simulink model "control_model_4"  (R2025b)
settings: Solver=VariableStepAuto  StartTime=0.0  StopTime=300  RelTol=1e-3
values from neighbouring files (symbols this model uses):
  Am = [0 1; -wn^2 -2*zeta*wn]    [Script.m]    (also in main_v2.m = [0 1 0 0; -walpha^2 -2*zeta_alpha*walpha 0 0; 0 0 0 1; 0 0 -; script_plane.m; script_v2.m)
  B = [0; -thrust*static_margin/Iy]    [Script.m]    (also in main_v2.m = [0; Cm_delta/Iy; 0; 0]; script_plane.m = [0; Cm_delta/Iy]; script_v2.m)
  Bm = [0; wn^2]    [Script.m]    (also in main_v2.m = [0; walpha^2; 0; 0]; script_plane.m; script_v2.m)
  c = 3.2    [main_v2.m]    (also in script_plane.m = 3.45)
  Cd0 = 0.02    [main_v2.m]
  Cl0 = 0.1    [main_v2.m]
  Cl_alpha = 5.7    [main_v2.m]
  Cm = [1 0; 0 1]    [Script.m]    (also in main_v2.m = eye(size(Am)); script_plane.m; script_v2.m)
  Cm_0 = -0.8    [main_v2.m]
  Cm_delta = -0.5    [main_v2.m]    (also in script_plane.m = -4.5)
  Cm_q = -12    [main_v2.m]    (also in script_plane.m = -8)
  delta_max = deg2rad(25)    [main_v2.m]    (also in script_plane.m)
  desired_aoa = deg2rad(45)    [main_v2.m]    (also in script_plane.m = deg2rad(20))
  Dm = [0;0]    [Script.m]    (also in main_v2.m = zeros(4, 1); script_plane.m; script_v2.m)
  g = 9.81    [Script.m]    (also in main_v2.m; script_v2.m)
  gain_e = 0    [main_v2.m]    (also in script_plane.m = 5000)
  gain_r = 300    [main_v2.m]    (also in script_plane.m = 50000)
  gain_x = 200    [main_v2.m]    (also in script_plane.m = 50000)
  Iy = 5    [Script.m]    (also in main_v2.m = 160000; script_plane.m = 70000; script_v2.m)
  K = 1/2 *rho * S *c    (= 58.8)    [main_v2.m]    (also in script_plane.m = 1908126.5175)
  k_d1 = 0.045    [main_v2.m]
  k_d2 = 0.08    [main_v2.m]
  kl = 3    [main_v2.m]
  Kr = wn^2/(-thrust*static_margin/Iy)    (= -0.0208333333333)    [Script.m]    (also in main_v2.m = 0; script_plane.m = -0.18; script_v2.m)
  Kx = ((Am-A)/B.').'    [Script.m]    (also in main_v2.m = [0 0 0 0]; script_plane.m = [0.21 0.05]; script_v2.m)
  mass = 15    [Script.m]    (also in main_v2.m = 9000; script_plane.m = 12000; script_v2.m)
  P = lyap(Am',Q)    [Script.m]    (also in main_v2.m; script_plane.m)
  rate_of_change = 4    [main_v2.m]
  rate_of_freeze_angle = 0.8    [main_v2.m]
  rate_of_freeze_rate = 2    [main_v2.m]
  rho = 1.225    [main_v2.m]    (also in script_plane.m)
  S = 30    [main_v2.m]    (also in script_plane.m = 27.87)
  sigma_r = 0.0003    [main_v2.m]    (also in script_plane.m = 1e-05)
  sigma_w = 0.0003    [main_v2.m]    (also in script_plane.m = 1e-05)
  sigma_x = 0.0003    [main_v2.m]    (also in script_plane.m = 1e-05)
  speed = 180    [main_v2.m]    (also in script_plane.m)
  thrust = 6000    [Script.m]    (also in main_v2.m = 160000; script_v2.m)
  W = [0 0 0 0]    [main_v2.m]
libraries: simulink_extras x17, simulink x2, slctrl_adaptive x1
settings Model: Creator=marti  LastModifiedBy=marti
settings SolverCC: ZeroCrossAlgorithm=Adaptive
settings DebuggingCC: IgnoredZcDiagnostic=none

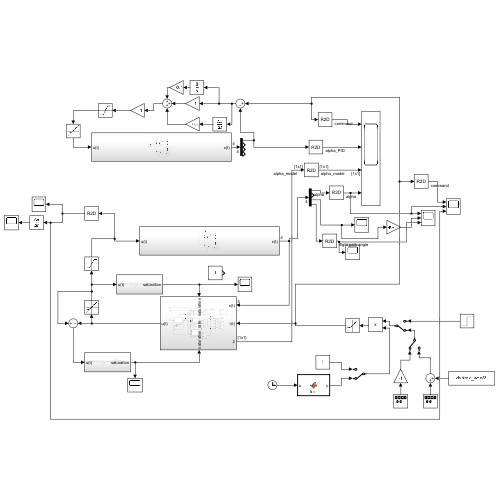
[thumbnail: Simulink's stored preview of the top-level diagram]
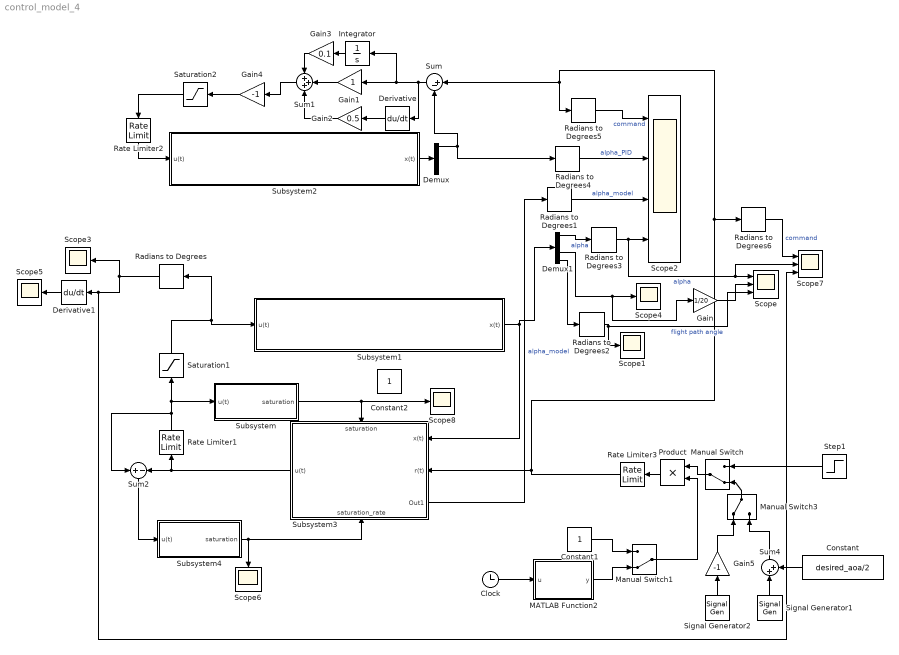
== system control_model_4 ==
  Clock : Clock
  Constant : Constant  Value=desired_aoa/2
  Constant1 : Constant
  Constant2 : Constant
  Demux : Demux
  Demux1 : Demux
  Derivative : Derivative
  Derivative1 : Derivative
  Gain : Gain  Gain=1/20
  Gain1 : Gain
  Gain2 : Gain  Gain=0.5
  Gain3 : Gain  Gain=0.1
  Gain4 : Gain  Gain=-1
  Gain5 : Gain  Gain=-1
  Integrator : Integrator
  MATLAB Function2 : MATLAB Function  TreatAsAtomicUnit=on
  Manual Switch : ManualSwitch  CurrentSetting=0
  Manual Switch1 : ManualSwitch  CurrentSetting=0
  Manual Switch3 : ManualSwitch
  Product : Product
  Radians to Degrees{,1..6} (7 alike) : simulink_extras/Transformations/Radians to Degrees
  Rate Limiter1 : RateLimiter  RisingSlewLimit=deg2rad(60)  FallingSlewLimit=-deg2rad(60)  SampleTimeMode=inherited
  Rate Limiter2 : RateLimiter  RisingSlewLimit=deg2rad(60)  FallingSlewLimit=-deg2rad(60)  SampleTimeMode=inherited
  Rate Limiter3 : RateLimiter  RisingSlewLimit=deg2rad(50)  FallingSlewLimit=-deg2rad(50)  SampleTimeMode=inherited
  Saturation1 : Saturate  UpperLimit=delta_max  LowerLimit=-delta_max  ZeroCross=off
  Saturation2 : Saturate  UpperLimit=delta_max  LowerLimit=-delta_max  ZeroCross=off
  Scope : Scope  NumInputPorts=3
      settings: ActiveDisplayYMinimum=-57.288074409345953  ActiveDisplayYMaximum=57.41030738577799  DataLoggingVariableName=ScopeData3
  Scope{1,3..6,8} (6 alike) : Scope
      Scope1 settings: ActiveDisplayYMinimum=-6.2979573477285218  ActiveDisplayYMaximum=52.72463637167975  DataLoggingVariableName=ScopeData2
      Scope3 settings: ActiveDisplayYMinimum=-31.25  ActiveDisplayYMaximum=31.25  DataLoggingVariableName=ScopeData16
      Scope4 settings: ActiveDisplayYMinimum=134.59247110443181  ActiveDisplayYMaximum=588.66776006011389  DataLoggingVariableName=ScopeData13
      Scope5 settings: ActiveDisplayYMinimum=-135.49485335885979  ActiveDisplayYMaximum=116.59818871809171  DataLoggingVariableName=ScopeData17
      Scope6 settings: ActiveDisplayYMinimum=-0.12499999999999997  ActiveDisplayYMaximum=1.125  DataLoggingVariableName=ScopeData12
      Scope8 settings: ActiveDisplayYMinimum=-0.1187909152069436  ActiveDisplayYMaximum=1.1243100993994897  DataLoggingVariableName=ScopeData18
  Scope2 : Scope  NumInputPorts=4
      settings: ActiveDisplayYMinimum=-78.018833846939785  ActiveDisplayYMaximum=59.661096228054994  DataLoggingVariableName=ScopeData15
  Scope7 : Scope  NumInputPorts=3
      settings: ActiveDisplayYMinimum=-1  ActiveDisplayYMaximum=1  DataLoggingVariableName=ScopeData14
  Signal Generator1 : SignalGenerator  WaveForm=square  Amplitude=desired_aoa/2  Frequency=0.1  Units=rad/sec
  Signal Generator2 : SignalGenerator  WaveForm=square  Amplitude=desired_aoa  Frequency=0.1  Units=rad/sec
  Step1 : Step  Time=31.3  After=desired_aoa  SampleTime=0
  Subsystem : Subsystem
  Subsystem1 : Subsystem
  Subsystem2 : Subsystem
  Subsystem3 : Subsystem
      settings: PortSchema="{\"entries\":[{\"content\":{\"sides\":[{\"content\":{\"connectorIds\":[\"Out2\",\"In1\",\"In2\"]},\"type\":\"ConnectorPlacement.EquallySpacedRectSide\",\"uuid\":\"2a5405b8-f474-466f-9064-f86b75893dd0\"},{\"content\":{\"connectorIds\":[\"Out1\"],\"side\":\"RIGHT\"},\"type\":\"ConnectorPlacement.EquallySpacedRectSide\",\"uuid\":\"ad673661-f4e9-494b-83cc-7452eec3fe31\"},{\"content\":{\"connectorIds\":[\"In3\"],\"side\":\"TOP\"},\"type\":\"ConnectorPlacement.EquallySpacedRectSide\",\"uuid\":\"21a76317-3288-4ff3-bd02-68708e86e3a8\"},{\"content\":{\"connectorIds\":[\"In4\"],\"side\":\"BOTTOM\"},\"type\":\"ConnectorPlacement.EquallySpacedRectSide\",\"uuid\":\"06318006-2373-43e5-8136-a784e8462fed\"}]},\"type\":\"ConnectorPlacement.EquallySpacedConnector\",\"uuid\":\"fc0ce599-928f-4c66-9629-0b98f2391e21\"}],\"packageUris\":[\"http://schema.mathworks.com/mf0/Connector/R2020b\"],\"version\":\"1.0\"}"
  Subsystem4 : Subsystem
  Sum : Sum  Inputs=|+-
  Sum1 : Sum  Inputs=+++
  Sum2 : Sum  Inputs=+|-
  Sum4 : Sum  Inputs=|++
  wires:
  Subsystem1/1(x(t)) -> Demux1/1, Subsystem3/2(x(t))
  Radians to Degrees3/1 -> Scope7/2, Scope/1, Scope2/4  "alpha"
  Radians to Degrees4/1 -> Scope2/2  "alpha_PID"
  Signal Generator1/1 -> Sum4/1
  Derivative1/1 -> Scope5/1
  Subsystem3/1(u(t)) -> Sum2/2, Rate Limiter1/1
  Subsystem4/1(saturation) -> Subsystem3/3(saturation_rate), Scope6/1
  Subsystem3/2(Out1) -> Radians to Degrees1/1  "alpha_model"
  Saturation1/1 -> Subsystem1/1(u(t)), Radians to Degrees/1
  Radians to Degrees1/1 -> Scope2/3  "alpha_model"
  Constant/1 -> Sum4/2
  Manual Switch3/1 -> Manual Switch/2
  Sum2/1 -> Subsystem4/1(u(t))
  Rate Limiter3/1 -> Subsystem3/1(r(t)), Radians to Degrees5/1, Sum/1, Radians to Degrees6/1
  Radians to Degrees5/1 -> Scope2/1  "command"
  Radians to Degrees/1 -> Scope7/3, Derivative1/1, Scope3/1
  Sum4/1 -> Manual Switch3/2
  Demux1/3 -> Gain/1, Scope4/1
  Radians to Degrees2/1 -> Scope1/1, Scope/3  "flight path angle"
  Clock/1 -> MATLAB Function2/1(u)
  Manual Switch/1 -> Product/1
  Product/1 -> Rate Limiter3/1
  Demux1/1 -> Radians to Degrees3/1  "alpha"
  Demux1/4 -> Radians to Degrees2/1
  Step1/1 -> Manual Switch/1
  Constant1/1 -> Manual Switch1/1
  MATLAB Function2/1(y) -> Manual Switch1/2
  Manual Switch1/1 -> Product/2
  Gain/1 -> Scope/2
  Subsystem/1(saturation) -> Scope8/1, Subsystem3/4(saturation)
  Sum/1 -> Derivative/1, Integrator/1, Gain1/1
  Subsystem2/1(x(t)) -> Demux/1
  Demux/1 -> Sum/2, Radians to Degrees4/1
  Gain1/1 -> Sum1/2
  Gain2/1 -> Sum1/3
  Integrator/1 -> Gain3/1
  Gain3/1 -> Sum1/1
  Derivative/1 -> Gain2/1
  Gain4/1 -> Saturation2/1
  Sum1/1 -> Gain4/1
  Saturation2/1 -> Rate Limiter2/1
  Rate Limiter2/1 -> Subsystem2/1(u(t))
  Rate Limiter1/1 -> Sum2/1, Saturation1/1, Subsystem/1(u(t))
  Signal Generator2/1 -> Gain5/1
  Gain5/1 -> Manual Switch3/1
  Radians to Degrees6/1 -> Scope7/1  "command"

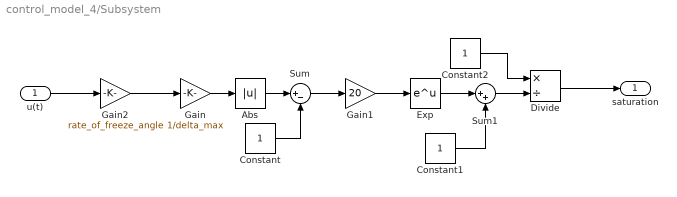
== system control_model_4/Subsystem ==
  u(t) : Inport
  Abs : Abs  SaturateOnIntegerOverflow=off
  Constant : Constant
  Constant1 : Constant
  Constant2 : Constant
  Divide : Product  Inputs=*/
  Exp : Math
  Gain : Gain  Gain=1/delta_max
  Gain1 : Gain  Gain=20
  Gain2 : Gain  Gain=rate_of_freeze_angle
  Sum : Sum  Inputs=|+-
  Sum1 : Sum  Inputs=|++
  saturation : Outport
  wires:
  Gain/1 -> Abs/1
  Abs/1 -> Sum/1
  Sum/1 -> Gain1/1
  Constant/1 -> Sum/2
  Gain1/1 -> Exp/1
  Exp/1 -> Sum1/1
  Constant1/1 -> Sum1/2
  Sum1/1 -> Divide/2
  Constant2/1 -> Divide/1
  Divide/1 -> saturation/1
  Gain2/1 -> Gain/1
  u(t)/1 -> Gain2/1

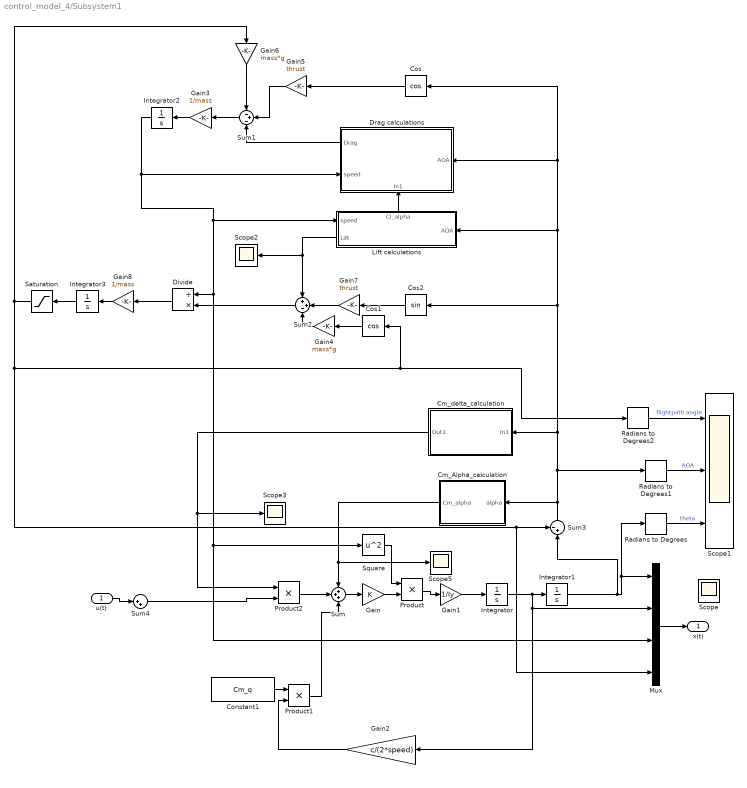
== system control_model_4/Subsystem1 ==
  u(t) : Inport
  Cm_Alpha_calculation : Subsystem
  Cm_delta_calculation : Subsystem
  Constant1 : Constant  Value=Cm_q
  Cos : Trigonometry  Operator=cos
  Cos1 : Trigonometry  Operator=cos
  Cos2 : Trigonometry
  Divide : Product  Inputs=/*
  Drag calculations : Subsystem
      settings: PortSchema="{\"entries\":[{\"content\":{\"sides\":[{\"content\":{\"connectorIds\":[\"Out1\",\"In1\"]},\"type\":\"ConnectorPlacement.EquallySpacedRectSide\",\"uuid\":\"d271dd9c-4b6b-493d-a484-ea343b2a7ea5\"},{\"content\":{\"connectorIds\":[\"In3\"],\"side\":\"RIGHT\"},\"type\":\"ConnectorPlacement.EquallySpacedRectSide\",\"uuid\":\"1c3a3b91-ae49-4f86-b72d-44481f1c47ea\"},{\"content\":{\"side\":\"TOP\"},\"type\":\"ConnectorPlacement.EquallySpacedRectSide\",\"uuid\":\"ad2c4e7a-6e16-439a-a8ce-91c789fc2dda\"},{\"content\":{\"connectorIds\":[\"In2\"],\"side\":\"BOTTOM\"},\"type\":\"ConnectorPlacement.EquallySpacedRectSide\",\"uuid\":\"1d27e3d2-8ebb-4b91-86b1-b9e0cbaba979\"}]},\"type\":\"ConnectorPlacement.EquallySpacedConnector\",\"uuid\":\"312dc24d-03ba-4f6d-95f4-f718ce8b3ee8\"}],\"packageUris\":[\"http://schema.mathworks.com/mf0/Connector/R2020b\"],\"version\":\"1.0\"}"
  Gain : Gain  Gain=K
  Gain1 : Gain  Gain=1/Iy
  Gain2 : Gain  Gain=c/(2*speed)
  Gain3 : Gain  Gain=1/mass
  Gain4 : Gain  Gain=mass*g
  Gain5 : Gain  Gain=thrust
  Gain6 : Gain  Gain=mass*g
  Gain7 : Gain  Gain=thrust
  Gain8 : Gain  Gain=1/mass
  Integrator : Integrator
  Integrator1 : Integrator
  Integrator2 : Integrator  InitialCondition=speed
  Integrator3 : Integrator
  Lift calculations : Subsystem
      settings: PortSchema="{\"entries\":[{\"content\":{\"sides\":[{\"content\":{\"connectorIds\":[\"In1\",\"Out2\"]},\"type\":\"ConnectorPlacement.EquallySpacedRectSide\",\"uuid\":\"5246f013-813c-4805-903b-98ed221a01a8\"},{\"content\":{\"connectorIds\":[\"In2\"],\"side\":\"RIGHT\"},\"type\":\"ConnectorPlacement.EquallySpacedRectSide\",\"uuid\":\"452079bc-9591-4c95-a88f-c45e08717f6a\"},{\"content\":{\"connectorIds\":[\"Out1\"],\"side\":\"TOP\"},\"type\":\"ConnectorPlacement.EquallySpacedRectSide\",\"uuid\":\"f365ba97-25c1-460b-8c6b-56706c8bd897\"}]},\"type\":\"ConnectorPlacement.EquallySpacedConnector\",\"uuid\":\"7294dbab-9b96-4a0b-a23a-2bd2309fe32e\"}],\"packageUris\":[\"http://schema.mathworks.com/mf0/Connector/R2020b\"],\"version\":\"1.0\"}"
  Mux : Mux
  Product : Product
  Product1 : Product
  Product2 : Product
  Radians to Degrees : simulink_extras/Transformations/Radians to Degrees
  Radians to Degrees1 : simulink_extras/Transformations/Radians to Degrees
  Radians to Degrees2 : simulink_extras/Transformations/Radians to Degrees
  Saturation : Saturate  UpperLimit=deg2rad(90)  LowerLimit=-deg2rad(90)
  Scope{,2..3,5} (4 alike) : Scope
      Scope settings: ActiveDisplayYMinimum=-0.01377254423088568  ActiveDisplayYMaximum=0.024994154646199356
      Scope2 settings: ActiveDisplayYMinimum=52037.469544787207  ActiveDisplayYMaximum=126455.77992982147  DataLoggingVariableName=ScopeData5
      Scope3 settings: ActiveDisplayYMinimum=-1  ActiveDisplayYMaximum=1  DataLoggingVariableName=ScopeData4
      Scope5 settings: ActiveDisplayYMinimum=-1  ActiveDisplayYMaximum=1  DataLoggingVariableName=ScopeData10
  Scope1 : Scope  NumInputPorts=3
      settings: ActiveDisplayYMinimum=-50.783545659916669  ActiveDisplayYMaximum=57.667479517478434
  Square : Math  Operator=square
  Sum : Sum  Inputs=+++
  Sum1 : Sum  Inputs=-+-
  Sum2 : Sum  Inputs=++-
  Sum3 : Sum  Inputs=-+|
  Sum4 : Sum  Inputs=|++
  x(t) : Outport
  wires:
  Product2/1 -> Sum/2
  Sum/1 -> Gain/1
  Gain1/1 -> Integrator/1
  Integrator/1 -> Mux/2, Gain2/1, Integrator1/1
  Constant1/1 -> Product1/1
  Product1/1 -> Sum/3
  Gain2/1 -> Product1/2
  Integrator1/1 -> Sum3/2, Mux/1, Radians to Degrees/1
  Cm_Alpha_calculation/1(Cm_alpha) -> Sum/1, Scope5/1
  Cm_delta_calculation/1(Out1) -> Product2/1, Scope3/1
  Lift calculations/2(Lift) -> Sum2/1, Scope2/1
  Lift calculations/1(Cl_alpha) -> Drag calculations/2(In1)
  Drag calculations/1(Drag) -> Sum1/3
  Cos/1 -> Gain5/1
  Gain5/1 -> Sum1/2
  Sum1/1 -> Gain3/1
  Gain3/1 -> Integrator2/1
  Integrator2/1 -> Drag calculations/1(speed), Lift calculations/1(speed), Mux/3, Square/1, Divide/1
  Cos1/1 -> Gain4/1
  Gain6/1 -> Sum1/1
  Gain4/1 -> Sum2/3
  Gain7/1 -> Sum2/2
  Cos2/1 -> Gain7/1
  Sum2/1 -> Divide/2
  Divide/1 -> Gain8/1
  Gain8/1 -> Integrator3/1
  Sum3/1 -> Radians to Degrees1/1, Cos2/1, Cos/1, Drag calculations/3(AOA), Lift calculations/2(AOA), Cm_delta_calculation/1(In1), Cm_Alpha_calculation/1(alpha)
  Gain/1 -> Product/2
  Product/1 -> Gain1/1
  Square/1 -> Product/1
  Radians to Degrees/1 -> Scope1/3  "theta"
  Radians to Degrees1/1 -> Scope1/2  "AOA"
  Radians to Degrees2/1 -> Scope1/1  "flightpath angle"
  Integrator3/1 -> Saturation/1
  Saturation/1 -> Mux/4, Sum3/1, Cos1/1, Radians to Degrees2/1, Gain6/1
  Mux/1 -> x(t)/1
  u(t)/1 -> Sum4/1
  Sum4/1 -> Product2/2

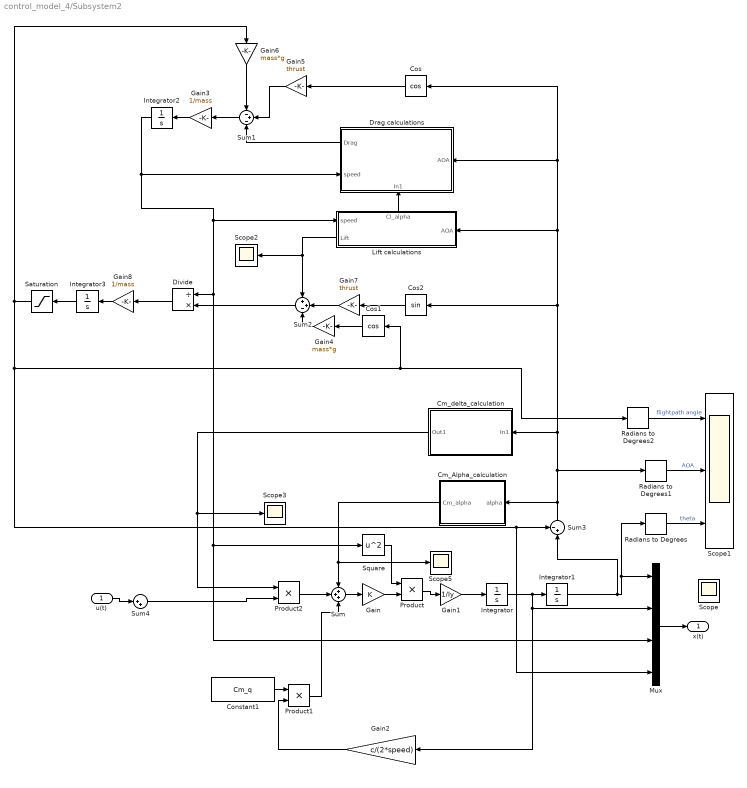
== system control_model_4/Subsystem2 ==
  u(t) : Inport
  Cm_Alpha_calculation : Subsystem
  Cm_delta_calculation : Subsystem
  Constant1 : Constant  Value=Cm_q
  Cos : Trigonometry  Operator=cos
  Cos1 : Trigonometry  Operator=cos
  Cos2 : Trigonometry
  Divide : Product  Inputs=/*
  Drag calculations : Subsystem
      settings: PortSchema="{\"entries\":[{\"content\":{\"sides\":[{\"content\":{\"connectorIds\":[\"Out1\",\"In1\"]},\"type\":\"ConnectorPlacement.EquallySpacedRectSide\",\"uuid\":\"d271dd9c-4b6b-493d-a484-ea343b2a7ea5\"},{\"content\":{\"connectorIds\":[\"In3\"],\"side\":\"RIGHT\"},\"type\":\"ConnectorPlacement.EquallySpacedRectSide\",\"uuid\":\"1c3a3b91-ae49-4f86-b72d-44481f1c47ea\"},{\"content\":{\"side\":\"TOP\"},\"type\":\"ConnectorPlacement.EquallySpacedRectSide\",\"uuid\":\"ad2c4e7a-6e16-439a-a8ce-91c789fc2dda\"},{\"content\":{\"connectorIds\":[\"In2\"],\"side\":\"BOTTOM\"},\"type\":\"ConnectorPlacement.EquallySpacedRectSide\",\"uuid\":\"1d27e3d2-8ebb-4b91-86b1-b9e0cbaba979\"}]},\"type\":\"ConnectorPlacement.EquallySpacedConnector\",\"uuid\":\"312dc24d-03ba-4f6d-95f4-f718ce8b3ee8\"}],\"packageUris\":[\"http://schema.mathworks.com/mf0/Connector/R2020b\"],\"version\":\"1.0\"}"
  Gain : Gain  Gain=K
  Gain1 : Gain  Gain=1/Iy
  Gain2 : Gain  Gain=c/(2*speed)
  Gain3 : Gain  Gain=1/mass
  Gain4 : Gain  Gain=mass*g
  Gain5 : Gain  Gain=thrust
  Gain6 : Gain  Gain=mass*g
  Gain7 : Gain  Gain=thrust
  Gain8 : Gain  Gain=1/mass
  Integrator : Integrator
  Integrator1 : Integrator
  Integrator2 : Integrator  InitialCondition=speed
  Integrator3 : Integrator
  Lift calculations : Subsystem
      settings: PortSchema="{\"entries\":[{\"content\":{\"sides\":[{\"content\":{\"connectorIds\":[\"In1\",\"Out2\"]},\"type\":\"ConnectorPlacement.EquallySpacedRectSide\",\"uuid\":\"5246f013-813c-4805-903b-98ed221a01a8\"},{\"content\":{\"connectorIds\":[\"In2\"],\"side\":\"RIGHT\"},\"type\":\"ConnectorPlacement.EquallySpacedRectSide\",\"uuid\":\"452079bc-9591-4c95-a88f-c45e08717f6a\"},{\"content\":{\"connectorIds\":[\"Out1\"],\"side\":\"TOP\"},\"type\":\"ConnectorPlacement.EquallySpacedRectSide\",\"uuid\":\"f365ba97-25c1-460b-8c6b-56706c8bd897\"}]},\"type\":\"ConnectorPlacement.EquallySpacedConnector\",\"uuid\":\"7294dbab-9b96-4a0b-a23a-2bd2309fe32e\"}],\"packageUris\":[\"http://schema.mathworks.com/mf0/Connector/R2020b\"],\"version\":\"1.0\"}"
  Mux : Mux
  Product : Product
  Product1 : Product
  Product2 : Product
  Radians to Degrees : simulink_extras/Transformations/Radians to Degrees
  Radians to Degrees1 : simulink_extras/Transformations/Radians to Degrees
  Radians to Degrees2 : simulink_extras/Transformations/Radians to Degrees
  Saturation : Saturate  UpperLimit=deg2rad(90)  LowerLimit=-deg2rad(90)
  Scope{,2..3,5} (4 alike) : Scope
      Scope settings: ActiveDisplayYMinimum=-0.01377254423088568  ActiveDisplayYMaximum=0.024994154646199356
      Scope2 settings: ActiveDisplayYMinimum=52037.469544787207  ActiveDisplayYMaximum=126455.77992982147  DataLoggingVariableName=ScopeData5
      Scope3 settings: ActiveDisplayYMinimum=-1  ActiveDisplayYMaximum=1  DataLoggingVariableName=ScopeData4
      Scope5 settings: ActiveDisplayYMinimum=-1  ActiveDisplayYMaximum=1  DataLoggingVariableName=ScopeData10
  Scope1 : Scope  NumInputPorts=3
      settings: ActiveDisplayYMinimum=-50.783545659916669  ActiveDisplayYMaximum=57.667479517478434
  Square : Math  Operator=square
  Sum : Sum  Inputs=+++
  Sum1 : Sum  Inputs=-+-
  Sum2 : Sum  Inputs=++-
  Sum3 : Sum  Inputs=-+|
  Sum4 : Sum  Inputs=|++
  x(t) : Outport
  wires:
  Product2/1 -> Sum/2
  Sum/1 -> Gain/1
  Gain1/1 -> Integrator/1
  Integrator/1 -> Mux/2, Gain2/1, Integrator1/1
  Constant1/1 -> Product1/1
  Product1/1 -> Sum/3
  Gain2/1 -> Product1/2
  Integrator1/1 -> Sum3/2, Mux/1, Radians to Degrees/1
  Cm_Alpha_calculation/1(Cm_alpha) -> Sum/1, Scope5/1
  Cm_delta_calculation/1(Out1) -> Product2/1, Scope3/1
  Lift calculations/2(Lift) -> Sum2/1, Scope2/1
  Lift calculations/1(Cl_alpha) -> Drag calculations/2(In1)
  Drag calculations/1(Drag) -> Sum1/3
  Cos/1 -> Gain5/1
  Gain5/1 -> Sum1/2
  Sum1/1 -> Gain3/1
  Gain3/1 -> Integrator2/1
  Integrator2/1 -> Drag calculations/1(speed), Lift calculations/1(speed), Mux/3, Square/1, Divide/1
  Cos1/1 -> Gain4/1
  Gain6/1 -> Sum1/1
  Gain4/1 -> Sum2/3
  Gain7/1 -> Sum2/2
  Cos2/1 -> Gain7/1
  Sum2/1 -> Divide/2
  Divide/1 -> Gain8/1
  Gain8/1 -> Integrator3/1
  Sum3/1 -> Radians to Degrees1/1, Cos2/1, Cos/1, Drag calculations/3(AOA), Lift calculations/2(AOA), Cm_delta_calculation/1(In1), Cm_Alpha_calculation/1(alpha)
  Gain/1 -> Product/2
  Product/1 -> Gain1/1
  Square/1 -> Product/1
  Radians to Degrees/1 -> Scope1/3  "theta"
  Radians to Degrees1/1 -> Scope1/2  "AOA"
  Radians to Degrees2/1 -> Scope1/1  "flightpath angle"
  Integrator3/1 -> Saturation/1
  Saturation/1 -> Mux/4, Sum3/1, Cos1/1, Radians to Degrees2/1, Gain6/1
  Mux/1 -> x(t)/1
  u(t)/1 -> Sum4/1
  Sum4/1 -> Product2/2

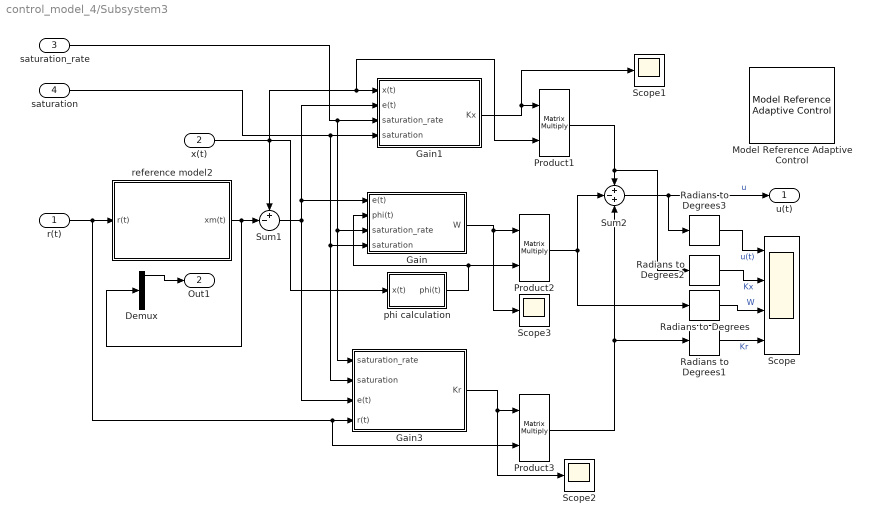
== system control_model_4/Subsystem3 ==
  r(t) : Inport
  x(t) : Inport  Port=2
  saturation_rate : Inport  Port=3
  saturation : Inport  Port=4
  Demux : Demux
  Gain : Subsystem
  Gain1 : Subsystem
  Gain3 : Subsystem
  Model Reference Adaptive Control : slctrl_adaptive/Model Reference Adaptive Control  selectType=Direct  A=0  B=1  Ahat=0  ALrEnable=on  gamma_a=1  ALrEnableMod=on  Bhat=1  BLrEnable=on  gamma_b=1  BLrEnableMod=on  externalKtauEnable=off  k_tau=-1  estParamOutput=off  Am=-1  Bm=1  kx=0  FBLrEnable=on  gamma_kx=1  FBLrEnableMod=on  kr=0  FFLrEnable=on  gamma_kr=1  FFLrEnableMod=on  AdaptEnable=on  gamma=1  WLrEnableMod=on  Q=1  FeatureTypeOptions=State  shlHiddenLayerSize=10  gamma_V=0.1  nCen=20  cSpanMin=-1  cSpanMax=1  cSig=5  adaptiveCntrlOutport=off  modChoice=None  sigma_val=0.1  DiscreteEnable=off  Ts=0.05  IntegrationMethods=Forward Euler
      settings: LibrarySourceBlock=slctrlblks/Adaptive Control/Model Reference Adaptive Control
  Product1 : Product  Multiplication=Matrix(*)
  Product2 : Product  Multiplication=Matrix(*)
  Product3 : Product  Multiplication=Matrix(*)
  Radians to Degrees{,1..3} (4 alike) : simulink_extras/Transformations/Radians to Degrees
  Scope : Scope  NumInputPorts=4
      settings: ActiveDisplayYMinimum=-28.327459556530236  ActiveDisplayYMaximum=38.233456732703587  DataLoggingVariableName=ScopeData6
  Scope1 : Scope
      settings: ActiveDisplayYMinimum=-3.3414581881686283E-5  ActiveDisplayYMaximum=0.00026683432418941894  DataLoggingVariableName=ScopeData7
  Scope2 : Scope
      settings: ActiveDisplayYMinimum=-1.0515209486810562E-6  ActiveDisplayYMaximum=6.83789903481209E-6  DataLoggingVariableName=ScopeData8
  Scope3 : Scope
      settings: ActiveDisplayYMinimum=-1  ActiveDisplayYMaximum=1  DataLoggingVariableName=ScopeData9
  Sum1 : Sum  Inputs=+-|
  Sum2 : Sum  Inputs=+-+
  phi calculation : Subsystem
  reference model2 : Subsystem  TreatAsAtomicUnit=on
  u(t) : Outport
  Out1 : Outport  Port=2
  wires:
  r(t)/1 -> Product3/2, Gain3/4(r(t)), reference model2/1(r(t))
  reference model2/1(xm(t)) -> Sum1/2, Demux/1
  x(t)/1 -> phi calculation/1(x(t)), Gain1/1(x(t)), Product1/2, Sum1/1
  Sum1/1 -> Gain/1(e(t)), Gain1/2(e(t)), Gain3/3(e(t))
  Product1/1 -> Radians to Degrees2/1, Sum2/1
  Gain/1(W) -> Scope3/1, Product2/1
  Gain1/1(Kx) -> Scope1/1, Product1/1
  Gain3/1(Kr) -> Scope2/1, Product3/1
  Product3/1 -> Sum2/3, Radians to Degrees1/1
  Product2/1 -> Radians to Degrees/1, Sum2/2
  Radians to Degrees2/1 -> Scope/2  "Kx"
  Radians to Degrees/1 -> Scope/3  "W"
  Radians to Degrees1/1 -> Scope/4  "Kr"
  Sum2/1 -> Radians to Degrees3/1, u(t)/1  "u"
  Radians to Degrees3/1 -> Scope/1  "u(t)"
  saturation_rate/1 -> Gain1/3(saturation_rate), Gain3/1(saturation_rate), Gain/3(saturation_rate)
  saturation/1 -> Gain3/2(saturation), Gain/4(saturation), Gain1/4(saturation)
  phi calculation/1(phi(t)) -> Gain/2(phi(t)), Product2/2
  Demux/1 -> Out1/1

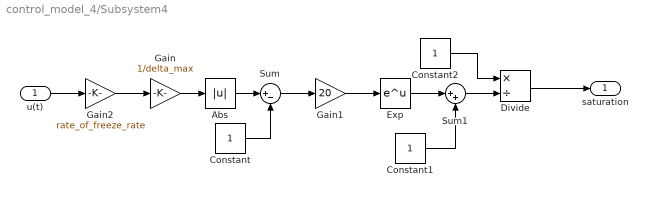
== system control_model_4/Subsystem4 ==
  u(t) : Inport
  Abs : Abs  SaturateOnIntegerOverflow=off
  Constant : Constant
  Constant1 : Constant
  Constant2 : Constant
  Divide : Product  Inputs=*/
  Exp : Math
  Gain : Gain  Gain=1/delta_max
  Gain1 : Gain  Gain=20
  Gain2 : Gain  Gain=rate_of_freeze_rate
  Sum : Sum  Inputs=|+-
  Sum1 : Sum  Inputs=|++
  saturation : Outport
  wires:
  Gain/1 -> Abs/1
  Abs/1 -> Sum/1
  Sum/1 -> Gain1/1
  Constant/1 -> Sum/2
  Gain1/1 -> Exp/1
  Exp/1 -> Sum1/1
  Constant1/1 -> Sum1/2
  Sum1/1 -> Divide/2
  Constant2/1 -> Divide/1
  Divide/1 -> saturation/1
  Gain2/1 -> Gain/1
  u(t)/1 -> Gain2/1

== system control_model_4/Subsystem1/Cm_Alpha_calculation ==
  alpha : Inport
  Constant : Constant
  Constant1 : Constant
  Divide : Product  Inputs=*/
  Gain : Gain  Gain=1/deg2rad(15)
  Gain7 : Gain  Gain=Cm_0
  Product : Product
  Scope5 : Scope
      settings: ActiveDisplayYMinimum=-1  ActiveDisplayYMaximum=1  DataLoggingVariableName=ScopeData11
  Square : Math  Operator=square
  Sum : Sum  Inputs=|++
  Cm_alpha : Outport
  wires:
  Product/1 -> Cm_alpha/1
  Gain7/1 -> Scope5/1, Product/2
  Gain/1 -> Square/1
  alpha/1 -> Gain/1, Product/1
  Square/1 -> Sum/1
  Constant/1 -> Sum/2
  Sum/1 -> Divide/2
  Divide/1 -> Gain7/1
  Constant1/1 -> Divide/1

== system control_model_4/Subsystem1/Cm_delta_calculation ==
  In1 : Inport
  Constant11 : Constant  Value=Cm_delta
  Constant2 : Constant
  Divide : Product  Inputs=/*
  Gain5 : Gain  Gain=rate_of_change
  Square : Math  Operator=square
  Sum4 : Sum  Inputs=++|
  Out1 : Outport
  wires:
  Gain5/1 -> Sum4/2
  Constant2/1 -> Sum4/1
  Divide/1 -> Out1/1
  Sum4/1 -> Divide/1
  Constant11/1 -> Divide/2
  Square/1 -> Gain5/1
  In1/1 -> Square/1

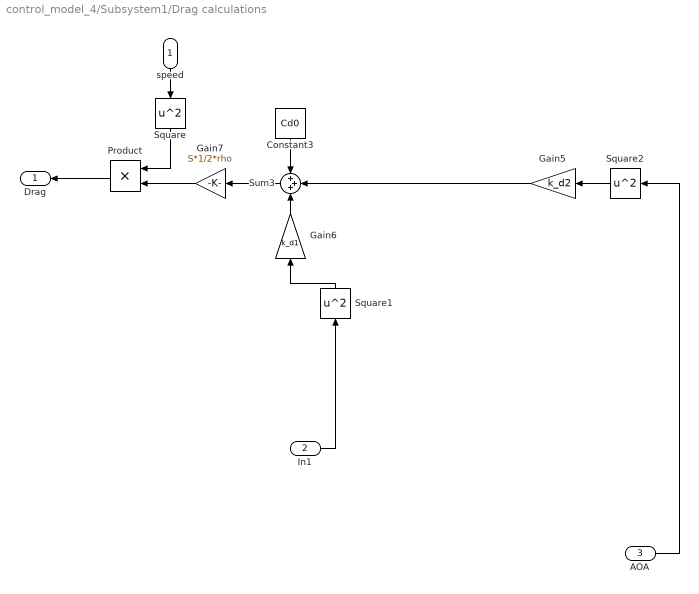
== system control_model_4/Subsystem1/Drag calculations ==
  speed : Inport
  In1 : Inport  Port=2
  AOA : Inport  Port=3
  Constant3 : Constant  Value=Cd0
  Gain5 : Gain  Gain=k_d2
  Gain6 : Gain  Gain=k_d1
  Gain7 : Gain  Gain=S*1/2*rho
  Product : Product
  Square : Math  Operator=square
  Square1 : Math  Operator=square
  Square2 : Math  Operator=square
  Sum3 : Sum  Inputs=+++
  Drag : Outport
  wires:
  Square1/1 -> Gain6/1
  Square2/1 -> Gain5/1
  Product/1 -> Drag/1
  Sum3/1 -> Gain7/1
  Gain6/1 -> Sum3/3
  Gain7/1 -> Product/2
  Constant3/1 -> Sum3/1
  Square/1 -> Product/1
  Gain5/1 -> Sum3/2
  AOA/1 -> Square2/1
  In1/1 -> Square1/1
  speed/1 -> Square/1

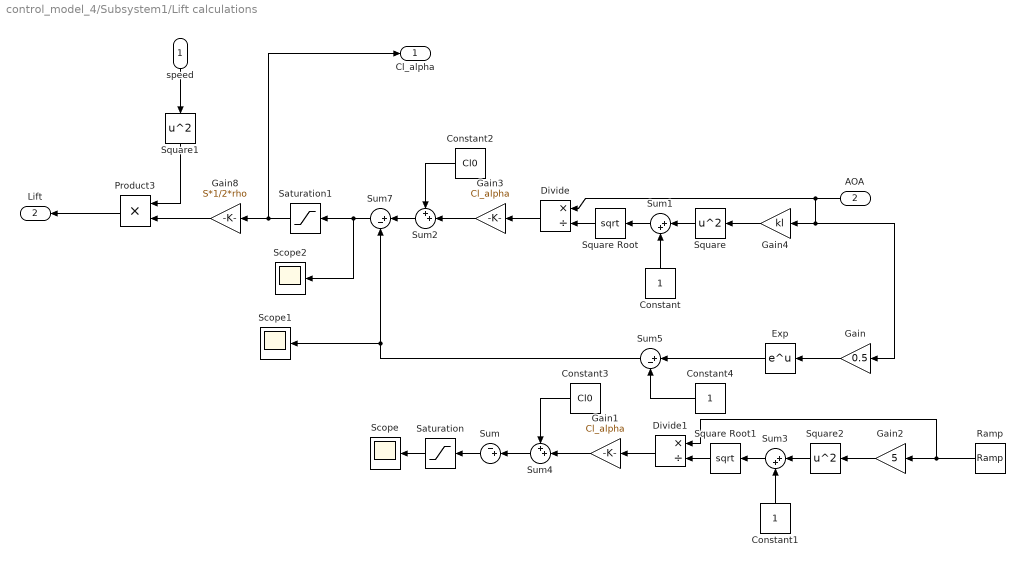
== system control_model_4/Subsystem1/Lift calculations ==
  speed : Inport
  AOA : Inport  Port=2
  Constant : Constant
  Constant1 : Constant
  Constant2 : Constant  Value=Cl0
  Constant3 : Constant  Value=Cl0
  Constant4 : Constant
  Divide : Product  Inputs=*/
  Divide1 : Product  Inputs=*/
  Exp : Math
  Gain : Gain  Gain=0.5
  Gain1 : Gain  Gain=Cl_alpha
  Gain2 : Gain  Gain=5
  Gain3 : Gain  Gain=Cl_alpha
  Gain4 : Gain  Gain=kl
  Gain8 : Gain  Gain=S*1/2*rho
  Product3 : Product
  Ramp : simulink/Sources/Ramp  slope=deg2rad(1)  start=0  InitialOutput=0
  Saturation : Saturate  UpperLimit=50  LowerLimit=0
  Saturation1 : Saturate  UpperLimit=50  LowerLimit=0
  Scope : Scope
      settings: ActiveDisplayYMinimum=-0.088318213479329374  ActiveDisplayYMaximum=0.79486392131396455  DataLoggingVariableName=ScopeData7
  Scope1 : Scope
      settings: ActiveDisplayYMinimum=-0.088318213479329374  ActiveDisplayYMaximum=0.79486392131396455  DataLoggingVariableName=ScopeData8
  Scope2 : Scope
      settings: ActiveDisplayYMinimum=0.082692694354211019  ActiveDisplayYMaximum=0.12337900982812083  DataLoggingVariableName=ScopeData9
  Square : Math  Operator=square
  Square Root : Sqrt
  Square Root1 : Sqrt
  Square1 : Math  Operator=square
  Square2 : Math  Operator=square
  Sum : Sum  Inputs=-+|
  Sum1 : Sum  Inputs=|++
  Sum2 : Sum  Inputs=++|
  Sum3 : Sum  Inputs=|++
  Sum4 : Sum  Inputs=++|
  Sum5 : Sum  Inputs=|+-
  Sum7 : Sum  Inputs=|+-
  Cl_alpha : Outport
  Lift : Outport  Port=2
  wires:
  Square/1 -> Sum1/1
  Square Root/1 -> Divide/2
  Gain3/1 -> Sum2/2
  Constant2/1 -> Sum2/1
  AOA/1 -> Divide/1, Gain/1, Gain4/1
  Gain4/1 -> Square/1
  Gain8/1 -> Product3/2
  Constant/1 -> Sum1/2
  Divide/1 -> Gain3/1
  Product3/1 -> Lift/1
  Sum1/1 -> Square Root/1
  Square1/1 -> Product3/1
  speed/1 -> Square1/1
  Divide1/1 -> Gain1/1
  Constant3/1 -> Sum4/1
  Square2/1 -> Sum3/1
  Square Root1/1 -> Divide1/2
  Gain1/1 -> Sum4/2
  Sum3/1 -> Square Root1/1
  Ramp/1 -> Divide1/1, Gain2/1
  Constant1/1 -> Sum3/2
  Gain2/1 -> Square2/1
  Sum4/1 -> Sum/2
  Exp/1 -> Sum5/1
  Constant4/1 -> Sum5/2
  Saturation/1 -> Scope/1
  Sum/1 -> Saturation/1
  Gain/1 -> Exp/1
  Sum2/1 -> Sum7/1
  Sum5/1 -> Scope1/1, Sum7/2
  Saturation1/1 -> Cl_alpha/1, Gain8/1
  Sum7/1 -> Scope2/1, Saturation1/1

== system control_model_4/Subsystem2/Cm_Alpha_calculation ==
  alpha : Inport
  Constant : Constant
  Constant1 : Constant
  Divide : Product  Inputs=*/
  Gain : Gain  Gain=1/deg2rad(15)
  Gain7 : Gain  Gain=Cm_0
  Product : Product
  Scope5 : Scope
      settings: ActiveDisplayYMinimum=-1  ActiveDisplayYMaximum=1  DataLoggingVariableName=ScopeData11
  Square : Math  Operator=square
  Sum : Sum  Inputs=|++
  Cm_alpha : Outport
  wires:
  Product/1 -> Cm_alpha/1
  Gain7/1 -> Scope5/1, Product/2
  Gain/1 -> Square/1
  alpha/1 -> Gain/1, Product/1
  Square/1 -> Sum/1
  Constant/1 -> Sum/2
  Sum/1 -> Divide/2
  Divide/1 -> Gain7/1
  Constant1/1 -> Divide/1

== system control_model_4/Subsystem2/Cm_delta_calculation ==
  In1 : Inport
  Constant11 : Constant  Value=Cm_delta
  Constant2 : Constant
  Divide : Product  Inputs=/*
  Gain5 : Gain  Gain=rate_of_change
  Square : Math  Operator=square
  Sum4 : Sum  Inputs=++|
  Out1 : Outport
  wires:
  Gain5/1 -> Sum4/2
  Constant2/1 -> Sum4/1
  Divide/1 -> Out1/1
  Sum4/1 -> Divide/1
  Constant11/1 -> Divide/2
  Square/1 -> Gain5/1
  In1/1 -> Square/1

== system control_model_4/Subsystem2/Drag calculations ==
  speed : Inport
  In1 : Inport  Port=2
  AOA : Inport  Port=3
  Constant3 : Constant  Value=Cd0
  Gain5 : Gain  Gain=k_d2
  Gain6 : Gain  Gain=k_d1
  Gain7 : Gain  Gain=S*1/2*rho
  Product : Product
  Square : Math  Operator=square
  Square1 : Math  Operator=square
  Square2 : Math  Operator=square
  Sum3 : Sum  Inputs=+++
  Drag : Outport
  wires:
  Square1/1 -> Gain6/1
  Square2/1 -> Gain5/1
  Product/1 -> Drag/1
  Sum3/1 -> Gain7/1
  Gain6/1 -> Sum3/3
  Gain7/1 -> Product/2
  Constant3/1 -> Sum3/1
  Square/1 -> Product/1
  Gain5/1 -> Sum3/2
  AOA/1 -> Square2/1
  In1/1 -> Square1/1
  speed/1 -> Square/1

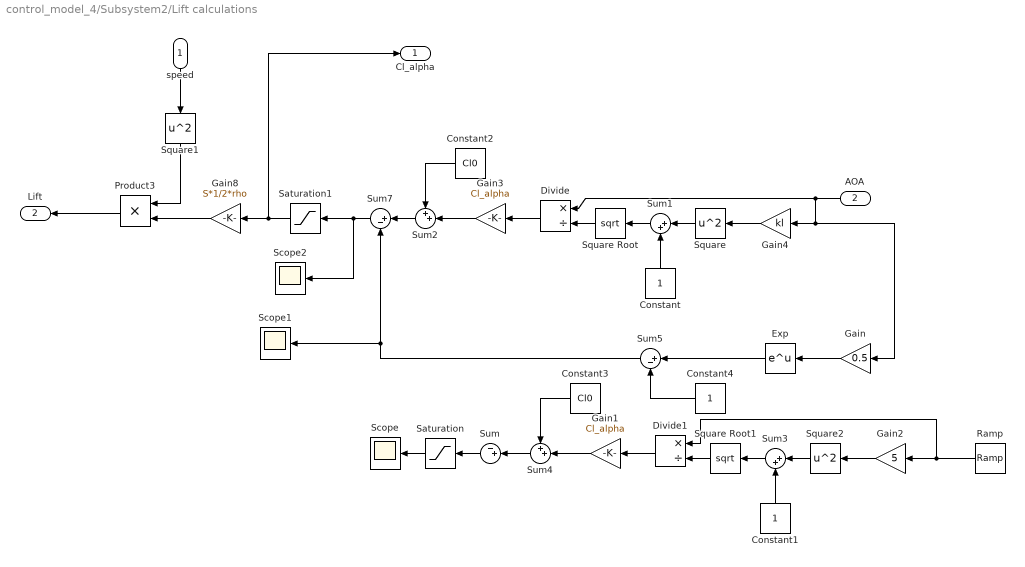
== system control_model_4/Subsystem2/Lift calculations ==
  speed : Inport
  AOA : Inport  Port=2
  Constant : Constant
  Constant1 : Constant
  Constant2 : Constant  Value=Cl0
  Constant3 : Constant  Value=Cl0
  Constant4 : Constant
  Divide : Product  Inputs=*/
  Divide1 : Product  Inputs=*/
  Exp : Math
  Gain : Gain  Gain=0.5
  Gain1 : Gain  Gain=Cl_alpha
  Gain2 : Gain  Gain=5
  Gain3 : Gain  Gain=Cl_alpha
  Gain4 : Gain  Gain=kl
  Gain8 : Gain  Gain=S*1/2*rho
  Product3 : Product
  Ramp : simulink/Sources/Ramp  slope=deg2rad(1)  start=0  InitialOutput=0
  Saturation : Saturate  UpperLimit=50  LowerLimit=0
  Saturation1 : Saturate  UpperLimit=50  LowerLimit=0
  Scope : Scope
      settings: ActiveDisplayYMinimum=-0.088318213479329374  ActiveDisplayYMaximum=0.79486392131396455  DataLoggingVariableName=ScopeData7
  Scope1 : Scope
      settings: ActiveDisplayYMinimum=-0.088318213479329374  ActiveDisplayYMaximum=0.79486392131396455  DataLoggingVariableName=ScopeData8
  Scope2 : Scope
      settings: ActiveDisplayYMinimum=0.082692694354211019  ActiveDisplayYMaximum=0.12337900982812083  DataLoggingVariableName=ScopeData9
  Square : Math  Operator=square
  Square Root : Sqrt
  Square Root1 : Sqrt
  Square1 : Math  Operator=square
  Square2 : Math  Operator=square
  Sum : Sum  Inputs=-+|
  Sum1 : Sum  Inputs=|++
  Sum2 : Sum  Inputs=++|
  Sum3 : Sum  Inputs=|++
  Sum4 : Sum  Inputs=++|
  Sum5 : Sum  Inputs=|+-
  Sum7 : Sum  Inputs=|+-
  Cl_alpha : Outport
  Lift : Outport  Port=2
  wires:
  Square/1 -> Sum1/1
  Square Root/1 -> Divide/2
  Gain3/1 -> Sum2/2
  Constant2/1 -> Sum2/1
  AOA/1 -> Divide/1, Gain/1, Gain4/1
  Gain4/1 -> Square/1
  Gain8/1 -> Product3/2
  Constant/1 -> Sum1/2
  Divide/1 -> Gain3/1
  Product3/1 -> Lift/1
  Sum1/1 -> Square Root/1
  Square1/1 -> Product3/1
  speed/1 -> Square1/1
  Divide1/1 -> Gain1/1
  Constant3/1 -> Sum4/1
  Square2/1 -> Sum3/1
  Square Root1/1 -> Divide1/2
  Gain1/1 -> Sum4/2
  Sum3/1 -> Square Root1/1
  Ramp/1 -> Divide1/1, Gain2/1
  Constant1/1 -> Sum3/2
  Gain2/1 -> Square2/1
  Sum4/1 -> Sum/2
  Exp/1 -> Sum5/1
  Constant4/1 -> Sum5/2
  Saturation/1 -> Scope/1
  Sum/1 -> Saturation/1
  Gain/1 -> Exp/1
  Sum2/1 -> Sum7/1
  Sum5/1 -> Scope1/1, Sum7/2
  Saturation1/1 -> Cl_alpha/1, Gain8/1
  Sum7/1 -> Scope2/1, Saturation1/1

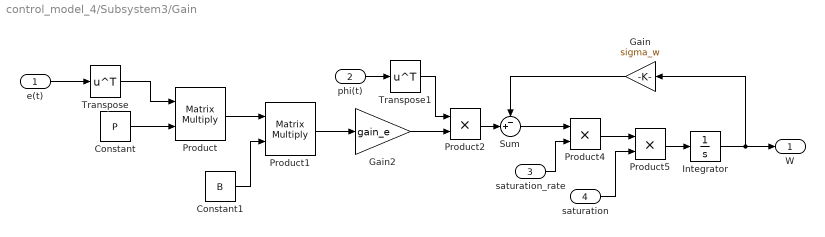
== system control_model_4/Subsystem3/Gain ==
  e(t) : Inport
  phi(t) : Inport  Port=2
  saturation_rate : Inport  Port=3
  saturation : Inport  Port=4
  Constant : Constant  Value=P  VectorParams1D=off
  Constant1 : Constant  Value=B  VectorParams1D=off
  Gain : Gain  Gain=sigma_w
  Gain2 : Gain  Gain=gain_e
  Integrator : Integrator  InitialCondition=W
  Product : Product  Multiplication=Matrix(*)
  Product1 : Product  Multiplication=Matrix(*)
  Product2 : Product
  Product4 : Product
  Product5 : Product
  Sum : Sum  Inputs=-+|
  Transpose : Math  Operator=transpose
  Transpose1 : Math  Operator=transpose
  W : Outport
  wires:
  Product1/1 -> Gain2/1
  Product/1 -> Product1/1
  Constant1/1 -> Product1/2
  Gain2/1 -> Product2/2
  e(t)/1 -> Transpose/1
  Constant/1 -> Product/2
  Transpose/1 -> Product/1
  Integrator/1 -> W/1, Gain/1
  phi(t)/1 -> Transpose1/1
  Transpose1/1 -> Product2/1
  Product2/1 -> Sum/2
  Gain/1 -> Sum/1
  saturation/1 -> Product5/2
  saturation_rate/1 -> Product4/2
  Sum/1 -> Product4/1
  Product4/1 -> Product5/1
  Product5/1 -> Integrator/1

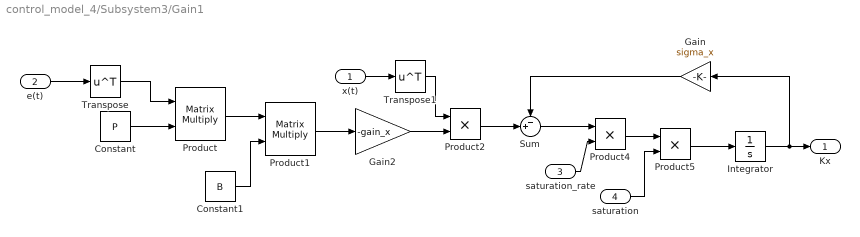
== system control_model_4/Subsystem3/Gain1 ==
  x(t) : Inport
  e(t) : Inport  Port=2
  saturation_rate : Inport  Port=3
  saturation : Inport  Port=4
  Constant : Constant  Value=P  VectorParams1D=off
  Constant1 : Constant  Value=B  VectorParams1D=off
  Gain : Gain  Gain=sigma_x
  Gain2 : Gain  Gain=-gain_x
  Integrator : Integrator  InitialCondition=Kx
  Product : Product  Multiplication=Matrix(*)
  Product1 : Product  Multiplication=Matrix(*)
  Product2 : Product
  Product4 : Product
  Product5 : Product
  Sum : Sum  Inputs=-+|
  Transpose : Math  Operator=transpose
  Transpose1 : Math  Operator=transpose
  Kx : Outport
  wires:
  Product1/1 -> Gain2/1
  Product/1 -> Product1/1
  Constant1/1 -> Product1/2
  Gain2/1 -> Product2/2
  e(t)/1 -> Transpose/1
  Constant/1 -> Product/2
  Transpose/1 -> Product/1
  Integrator/1 -> Gain/1, Kx/1
  x(t)/1 -> Transpose1/1
  Transpose1/1 -> Product2/1
  Product2/1 -> Sum/2
  Gain/1 -> Sum/1
  Sum/1 -> Product4/1
  Product4/1 -> Product5/1
  Product5/1 -> Integrator/1
  saturation_rate/1 -> Product4/2
  saturation/1 -> Product5/2

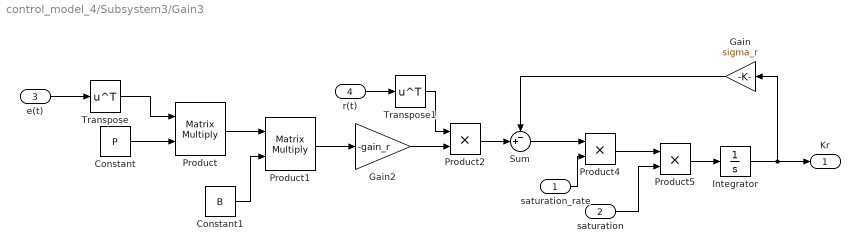
== system control_model_4/Subsystem3/Gain3 ==
  saturation_rate : Inport
  saturation : Inport  Port=2
  e(t) : Inport  Port=3
  r(t) : Inport  Port=4
  Constant : Constant  Value=P  VectorParams1D=off
  Constant1 : Constant  Value=B  VectorParams1D=off
  Gain : Gain  Gain=sigma_r
  Gain2 : Gain  Gain=-gain_r
  Integrator : Integrator  InitialCondition=Kr
  Product : Product  Multiplication=Matrix(*)
  Product1 : Product  Multiplication=Matrix(*)
  Product2 : Product
  Product4 : Product
  Product5 : Product
  Sum : Sum  Inputs=-+|
  Transpose : Math  Operator=transpose
  Transpose1 : Math  Operator=transpose
  Kr : Outport
  wires:
  Product1/1 -> Gain2/1
  Product/1 -> Product1/1
  Constant1/1 -> Product1/2
  Gain2/1 -> Product2/2
  Constant/1 -> Product/2
  Transpose/1 -> Product/1
  Integrator/1 -> Kr/1, Gain/1
  r(t)/1 -> Transpose1/1
  Transpose1/1 -> Product2/1
  Product2/1 -> Sum/2
  Gain/1 -> Sum/1
  e(t)/1 -> Transpose/1
  saturation/1 -> Product5/2
  saturation_rate/1 -> Product4/2
  Sum/1 -> Product4/1
  Product4/1 -> Product5/1
  Product5/1 -> Integrator/1

== system control_model_4/Subsystem3/phi calculation ==
  x(t) : Inport
  Constant2 : Constant  Value=0
  Demux1 : Demux
  Mux2 : Mux
  Product : Product
  Square : Math  Operator=square
  Sum : Sum  Inputs=|+-
  phi(t) : Outport
  wires:
  Sum/1 -> Product/1, Mux2/2
  Square/1 -> Product/2, Mux2/3
  Constant2/1 -> Mux2/1
  Product/1 -> Mux2/4
  Mux2/1 -> phi(t)/1
  x(t)/1 -> Demux1/1
  Demux1/4 -> Sum/2
  Demux1/1 -> Sum/1
  Demux1/3 -> Square/1

== system control_model_4/Subsystem3/reference model2 ==
  r(t) : Inport
  State-Space : StateSpace  A=Am  B=Bm  C=Cm  D=Dm  InitialCondition=[0;0;speed;0]
  xm(t) : Outport  PortDimensions=[4 1]
  wires:
  r(t)/1 -> State-Space/1
  State-Space/1 -> xm(t)/1

== matlab function control_model_4/MATLAB Function2 ==
  data: u input; y output
function y = fcn(u)
if u<30
    y=0;
else
    y=1;
end
